simulink model "Senario1"  (R2022a)
settings: Solver=VariableStepAuto  StartTime=0.0  StopTime=inf  RelTol=1e-3
undefined symbols (not defined in the file or in its folder): hys_max, hys_min, max_soc, min_soc
libraries: Assets x3, simulink x1
settings Model: PacingRate=10000  Creator=a.dehghan  LastModifiedBy=a.dehghan

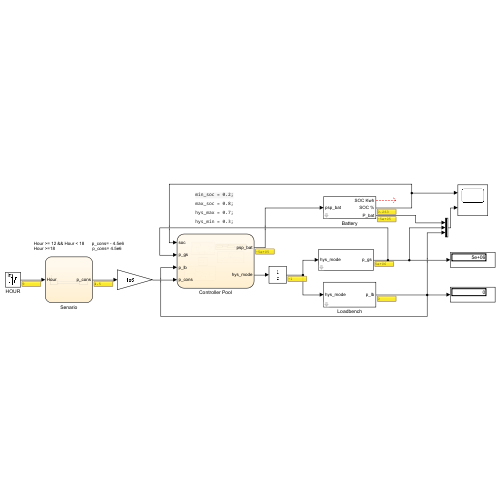
[thumbnail: Simulink's stored preview of the top-level diagram]
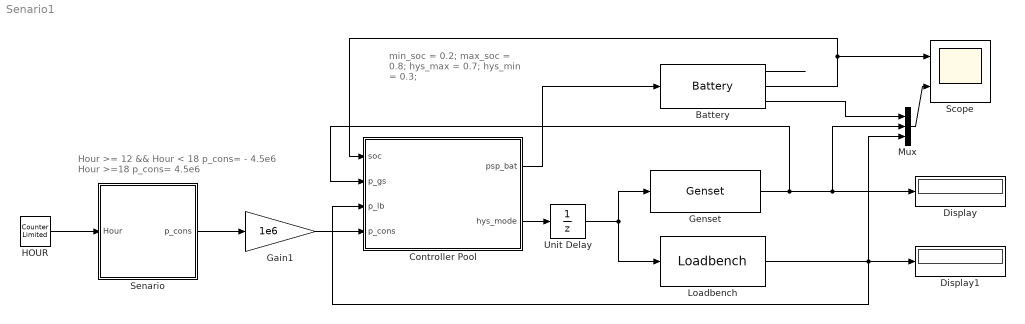
== system Senario1 ==
  note: Hour >= 12 && Hour < 18 p_cons= - 4.5e6
      | Hour >=18 p_cons= 4.5e6
  note: min_soc = 0.2;
      | max_soc = 0.8;
      | hys_max = 0.7;
      | hys_min = 0.3;
  Battery : Assets/Battery  max_soc_limit=max_soc_limit  min_soc_limit=min_soc_limit  efficiency_discharge=efficiency_discharge  efficiency_charge=efficiency_charge  psp_bat=p  stock=stock  ini_state_of_charge=ini_state_of_charge
      settings: SourceProductName=My Library
  Controller Pool : Stateflow chart  TreatAsAtomicUnit=on
  Display : Display
  Display1 : Display
  Gain1 : Gain  Gain=1e6
  Genset : Assets/Genset  hys_mode=[0 -1]  p_max_gs=p_max_gs  rising_slew_rate=rising_slew_rate  falling_slew_rate=falling_slew_rate
      link override GS dynamics/Rate Limiter: RisingSlewLimit=rising_slew_rate*1e6/60  FallingSlewLimit=falling_slew_rate*1e6/60
      settings: SourceProductName=My Library
  HOUR : simulink/Sources/Counter Limited  uplimit=24  tsamp=3600
  Loadbench : Assets/Loadbench  hys_mode=[0 1]  p_max_lb=p_max_lb
      settings: SourceProductName=My Library
  Mux : Mux  Inputs=3
  Scope : Scope  NumInputPorts=2
  Senario : Stateflow chart  TreatAsAtomicUnit=on
  Unit Delay : UnitDelay  HasFrameUpgradeWarning=on
  wires:
  Controller Pool/2(hys_mode) -> Unit Delay/1
  Battery/2 -> Scope/1, Controller Pool/1(soc)
  Loadbench/1 -> Mux/3, Display1/1, Controller Pool/3(p_lb)
  Controller Pool/1(psp_bat) -> Battery/1
  HOUR/1 -> Senario/1(Hour)
  Genset/1 -> Controller Pool/2(p_gs), Mux/2, Display/1
  Unit Delay/1 -> Genset/1, Loadbench/1
  Senario/1(p_cons) -> Gain1/1
  Mux/1 -> Scope/2
  Gain1/1 -> Controller Pool/4(p_cons)
  Battery/3 -> Mux/1
  Battery/1 -> ?

== stateflow chart Senario1/Controller Pool ==
  state ? [commented out]
    state Battery1 [commented out]
      entry : p_cons = psp_bat;
      during :
      psp_gs = 0;
      psp_lb = 0;
    state Genset1 [commented out]
      entry : p_cons = psp_gs;
      during :
      psp_lb = 0;
      psp_bat = 0;
    state Loadbench1 [commented out]
      entry : p_cons = psp_lb
      during :
      psp_gs = 0;
      psp_bat = 0;
    ?.Battery1 -> Genset1 [commented out] : [SOC < min_soc && p_cons >=0]
    Genset1 -> ?.Battery1 [commented out] : [min_soc < SOC < max_soc]
    Genset1 -> Loadbench1 [commented out] : [SOC > max_soc && p_cons <=0]
    Loadbench1 -> Genset1 [commented out]
    Loadbench1 -> ?.Battery1 [commented out] : [min_soc < SOC < max_soc]
    ?.Battery1 -> Loadbench1 [commented out]
  state Hysteresis_mode
    state Mode___1
      en : hys_mode = -1;
      du : psp_bat = p_cons - p_lb - p_gs;
    state Mode_0
      en : hys_mode = 0;
      du : psp_bat = p_cons - p_lb - p_gs;
    state Mode_1
      en : hys_mode = 1;
      du : psp_bat = p_cons - p_lb - p_gs;
    (default) -> Mode_0
    Mode_0 -> Mode___1 [order 2] : [soc <= min_soc]
    Mode_0 -> Mode_1 [order 1] : [soc >= max_soc]
    Mode___1 -> Mode_0 : [soc >= hys_min]
    Mode_1 -> Mode_0 : [soc <= hys_max]
  state Dispatcher1 [commented out]
    state Battery1 [commented out]
      en :
      hys_mode = 0;
      p_cons = psp_bat;
    state LB_off [commented out]
      en : hys_mode = 0;
      du : p_cons = psp_bat;
    state LB_on [commented out]
      en : hys_mode = 1;
      du : p_cons = psp_lb;
    state GS_on [commented out]
      en : hys_mode = -1;
      du : p_cons = psp_gs;
    state GS_off [commented out]
      en : hys_mode = 0;
      du : p_cons = psp_bat;
    (default) -> Dispatcher1.Battery1 [commented out]
    Dispatcher1.Battery1 -> (junction 131) [commented out]
    (junction 131) -> GS_off [commented out] : [soc >= hys_min]
    (junction 131) -> LB_on [commented out] : [soc >= hys_max]
    (junction 131) -> GS_on [commented out] : [soc <= hys_min]
    (junction 131) -> LB_off [commented out] : [soc <= hys_max]
  state start_order [commented out]
    (default) -> (junction 74) [commented out] : % start_order
    (junction 74) -> (junction 75) [commented out] : [psp_gs > 0]
    (junction 74) -> (junction 76) [commented out] : {start_order = 0;}
    (junction 75) -> (junction 77) [commented out] : {start_order = 1;}
    (junction 77) -> (junction 76) [commented out]
    (junction 76) -> (junction 78) [commented out]
  state ? [commented out]
    state Battery [commented out]
      entry : p_cons = psp_bat;
      during :
      psp_gs = 0;
      psp_lb = 0;
    state Genset [commented out]
      entry : p_cons = psp_gs;
      during :
      psp_lb = 0;
      psp_bat = 0;
    state Loadbench [commented out]
      entry : p_cons = psp_lb
      during :
      psp_gs = 0;
      psp_bat = 0;
    (default) -> (junction 91) [commented out]
    (junction 91) -> Genset [commented out] : [SOC < min_soc && p_cons >=0]
    (junction 91) -> Loadbench [commented out] : [SOC > max_soc && p_cons <=0]
    (junction 91) -> Battery [commented out]
  data: soc input; p_gs input; p_lb input; psp_bat output; hys_mode output; p_cons input; min_soc parameter double; max_soc parameter double; hys_max parameter; hys_min parameter

== stateflow chart Senario1/Senario ==
  state decharge
    entry : p_cons = 4.5;
  state charge
    entry : p_cons = -4.5;
  (default) -> decharge
  decharge -> charge : [Hour >= 12 && Hour < 18]
  charge -> decharge : [Hour >=18]
  data: Hour input; p_cons output
